simulink model "QuadrotorSimulink_w_memory_cex"  (R2020a)
settings: Solver=FixedStepAuto  StartTime=0.0  StopTime=options.T_train  FixedStep=options.dt  RelTol=1e-6
undefined symbols (not defined in the file or in its folder): options, Quad
libraries: neural x179, simulink x2
(part 7 of 10)

== system QuadrotorSimulink_w_memory_cex/NN_cex_1/Layer 2/Delays 1 ==
  "p{2}" : Inport  PortDimensions=50
      mask Display: e = 0.06;c1 = [120 230 180]/255;c2 = ([120 230 180]+0)/(256+128);c3 = ([120 230 180]+128)/(256+128);patch([0 1 1 0],[0 0 1 1],c1);patch([0 1 1 1-e 1-e 0+e],[0 0 1 1-e 0+e 0+e],c2);patch([0 0 1 1-e 0+e 0+e],[0 1 1 1-e 1-e 0+e],c3);plot([0 1 1 0 0],[0 0 1 1 0]);
  mux : Mux  Inputs=1
      mask Display: e = 0.06;c1 = [120 150 230]/255;c2 = ([120 150 230]+0)/383;c3 = ([120 150 230]+128)/383;patch([0 1 1 0],[0 0 1 1],c1);patch([0 1 1 1-e 1-e 0+e],[0 0 1 1-e 0+e 0+e],c2);patch([0 0 1 1-e 0+e 0+e],[0 1 1 1-e 1-e 0+e],c3);plot([0 1 1 0 0],[0 0 1 1 0]);disp('Mux')
  "pd{2,1}" : Outport
      mask Display: e = 0.06;c1 = [120 230 180]/255;c2 = ([120 230 180]+0)/(256+128);c3 = ([120 230 180]+128)/(256+128);patch([0 1 1 0],[0 0 1 1],c1);patch([0 1 1 1-e 1-e 0+e],[0 0 1 1-e 0+e 0+e],c2);patch([0 0 1 1-e 0+e 0+e],[0 1 1 1-e 1-e 0+e],c3);plot([0 1 1 0 0],[0 0 1 1 0]);
  wires:
  "p{2}"/1 -> mux/1
  mux/1 -> "pd{2,1}"/1

== system QuadrotorSimulink_w_memory_cex/NN_cex_1/Layer 2/LW{2,1} ==
  "ad{2,1}" : Inport  PortDimensions=50
      mask Display: e = 0.06;c1 = [120 230 180]/255;c2 = ([120 230 180]+0)/(256+128);c3 = ([120 230 180]+128)/(256+128);patch([0 1 1 0],[0 0 1 1],c1);patch([0 1 1 1-e 1-e 0+e],[0 0 1 1-e 0+e 0+e],c2);patch([0 0 1 1-e 0+e 0+e],[0 1 1 1-e 1-e 0+e],c3);plot([0 1 1 0 0],[0 0 1 1 0]);
  "IW{2,1}(1,:)'" : Constant  Value=[0.0275538326993548347842999390877594123594462871551513671875;-0.00745565907937648618408754686015527113340795040130615234375;0.66611503175745812033170523136504925787448883056640625;0.05475901990521143958279282060175319202244281768798828125;0.344437347512224933954172456651576794683933258056640625;1.1839628141689633178401663826662115752696990966796875;0.3116370266453174497911504658986814320087432861328125;0.07730669959515919231751723827983369119465351104736328125;-0.363985665723801699034112289155018515884876251220703125;0.260799759684065268761088418614235706627368927001953125;0.5559553932390013386566351982764899730682373046875;0.5868367481176670619191781952395103871822357177734375;0.443563139631132641316213494064868427813053131103515625;-0.57228815188380888212549280069652013480663299560546875;-0.4472350845444739153577984325238503515720367431640625;0.52041429315349230222409460111521184444427490234375;-1.49514504832872052730863288161344826221466064453125;3.839025236523978090730224721482954919338226318359375;-0.83636038152684888391519280048669315874576568603515625;2.770261180892548136256436919211409986019134521484375;-2.174306258179516504469575011171400547027587890625;-0.63768806122568622019031181480386294424533843994140625;-0.10146963780517899433863959757218253798782825469970703125;0.12244143511869053086993375245583592914044857025146484375;-2.7050091972379295413020372507162392139434814453125;0.033883234388811377113537304239798686467111110687255859375;-1.937067165957502279383106724708341062068939208984375;-0.02434512567339365551877250481993542052805423736572265625;-1.3585729552029144340252742040320299565792083740234375;0.0223565759681883281795311546602533780969679355621337890625;-0.030950898275129201664412903483025729656219482421875;0.340697149373347663026123655072296969592571258544921875;-0.05852572617005451227623069598848815076053142547607421875;-0.231972598769883908698119512337143532931804656982421875;-0.95302626348313912441057027535862289369106292724609375;0.08234375105086695623146653133517247624695301055908203125;-0.366614535263205587600765511524514295160770416259765625;-0.321032350030504842752776539782644249498844146728515625;0.1386987404389075084765181600232608616352081298828125;-1.410332716268217101429627291508950293064117431640625;0.3876911750625680053161659088800661265850067138671875;-0.20222266246863485061879828208475373685359954833984375;-0.6371437523569614125307225549477152526378631591796875;3.0662912359927947392179703456349670886993408203125;-0.001165993548972417588605043903271507588215172290802001953125;0.2008899619525147672849385571680613793432712554931640625;-0.06816492792016214108397065274402848444879055023193359375;-0.424260573156220399670957021953654475510120391845703125;-0.69161791521699444995618932807701639831066131591796875;0.028596534180291795224082562754119862802326679229736328125]
      mask Display: e = 0.06;c1 = [120 150 230]/255;c2 = ([120 150 230]+0)/383;c3 = ([120 150 230]+128)/383;patch([0 1 1 0],[0 0 1 1],c1);patch([0 1 1 1-e 1-e 0+e],[0 0 1 1-e 0+e 0+e],c2);patch([0 0 1 1-e 0+e 0+e],[0 1 1 1-e 1-e 0+e],c3);plot([0 1 1 0 0],[0 0 1 1 0]);disp('weights');
  "IW{2,1}(2,:)'" : Constant  Value=[-0.280572973800752134554414851663750596344470977783203125;-0.06376826585401164371180726675447658635675907135009765625;-0.93476819146209855215801098893280141055583953857421875;0.72705169346194697954643970660981722176074981689453125;-0.172177864521904255834527930346666835248470306396484375;-0.140787185209432286203679041136638261377811431884765625;0.426538355970393634475357202973100356757640838623046875;-0.289439707405152291119776464256574399769306182861328125;-0.0824665563311895166709319937581312842667102813720703125;-0.8383003997238323012908267628517933189868927001953125;-0.01928863124126110883960194541941746138036251068115234375;-0.225346299303538888381126525928266346454620361328125;0.7088162243692701647290732580586336553096771240234375;1.0224955026034676652813004693598486483097076416015625;-0.35879716511517389943008993213879875838756561279296875;0.022128490980010594169069548797779134474694728851318359375;0.5357120852447663228446117500425316393375396728515625;-0.62766932055573765314449019570020027458667755126953125;1.61542308170520332311070887953974306583404541015625;0.775974994887877134175369064905680716037750244140625;1.049763304219808457418139369110576808452606201171875;1.6714230172228912163490122111397795379161834716796875;-0.78107883860749571791615153415477834641933441162109375;0.41180896979510694944082160873222164809703826904296875;0.078029770082390204066769001656211912631988525390625;0.157969748428506029380713471255148760974407196044921875;0.06930887115900750961028364827143377624452114105224609375;-0.25182521165821059039302554083405993878841400146484375;-0.0673017608440212578013728261794312857091426849365234375;0.388768076847751664626429146665032021701335906982421875;-1.9234002406917289906829182655201293528079986572265625;0.51762869081730322751155881633167155086994171142578125;-0.07740912225261709078694138952414505183696746826171875;-0.06686671100983776483417386771179735660552978515625;0.7419276245436730032878358542802743613719940185546875;-0.13904342636608524319541402292088605463504791259765625;1.6098178034438015426843548993929289281368255615234375;-0.517302732605810167143545186263509094715118408203125;0.67228285116788677466814760919078253209590911865234375;1.420489242967595711064632268971763551235198974609375;-0.434467130876859453092464491419377736747264862060546875;0.192631001166826132386944436802878044545650482177734375;-0.127809383809272814058743961140862666070461273193359375;1.26464664389063674576618723222054541110992431640625;0.1969724906545538833935182765344507060945034027099609375;0.62756673407505469963751920658978633582592010498046875;-0.26367215443778080352643655714928172528743743896484375;-0.576491403893907516930994461290538311004638671875;-0.1502827549216607661008993090945295989513397216796875;-0.01769473689937062221844144005444832146167755126953125]
      mask Display: e = 0.06;c1 = [120 150 230]/255;c2 = ([120 150 230]+0)/383;c3 = ([120 150 230]+128)/383;patch([0 1 1 0],[0 0 1 1],c1);patch([0 1 1 1-e 1-e 0+e],[0 0 1 1-e 0+e 0+e],c2);patch([0 0 1 1-e 0+e 0+e],[0 1 1 1-e 1-e 0+e],c3);plot([0 1 1 0 0],[0 0 1 1 0]);disp('weights');
  Mux : Mux  Inputs=2
      mask Display: e = 0.06;c1 = [120 150 230]/255;c2 = ([120 150 230]+0)/383;c3 = ([120 150 230]+128)/383;patch([0 1 1 0],[0 0 1 1],c1);patch([0 1 1 1-e 1-e 0+e],[0 0 1 1-e 0+e 0+e],c2);patch([0 0 1 1-e 0+e 0+e],[0 1 1 1-e 1-e 0+e],c3);plot([0 1 1 0 0],[0 0 1 1 0]);disp('Mux');
  dotprod1 : neural/Weight Functions/dotprod
  dotprod2 : neural/Weight Functions/dotprod
  "lz{2,1}" : Outport
      mask Display: e = 0.06;c1 = [120 230 180]/255;c2 = ([120 230 180]+0)/(256+128);c3 = ([120 230 180]+128)/(256+128);patch([0 1 1 0],[0 0 1 1],c1);patch([0 1 1 1-e 1-e 0+e],[0 0 1 1-e 0+e 0+e],c2);patch([0 0 1 1-e 0+e 0+e],[0 1 1 1-e 1-e 0+e],c3);plot([0 1 1 0 0],[0 0 1 1 0]);
  wires:
  "IW{2,1}(1,:)'"/1 -> dotprod1/1
  "ad{2,1}"/1 -> dotprod1/2, dotprod2/2
  dotprod1/1 -> Mux/1
  "IW{2,1}(2,:)'"/1 -> dotprod2/1
  dotprod2/1 -> Mux/2
  Mux/1 -> "lz{2,1}"/1

== system QuadrotorSimulink_w_memory_cex/NN_online/Layer 1/Delays 1 ==
  "p{1}" : Inport  PortDimensions=20
      mask Display: e = 0.06;c1 = [120 230 180]/255;c2 = ([120 230 180]+0)/(256+128);c3 = ([120 230 180]+128)/(256+128);patch([0 1 1 0],[0 0 1 1],c1);patch([0 1 1 1-e 1-e 0+e],[0 0 1 1-e 0+e 0+e],c2);patch([0 0 1 1-e 0+e 0+e],[0 1 1 1-e 1-e 0+e],c3);plot([0 1 1 0 0],[0 0 1 1 0]);
  mux : Mux  Inputs=1
      mask Display: e = 0.06;c1 = [120 150 230]/255;c2 = ([120 150 230]+0)/383;c3 = ([120 150 230]+128)/383;patch([0 1 1 0],[0 0 1 1],c1);patch([0 1 1 1-e 1-e 0+e],[0 0 1 1-e 0+e 0+e],c2);patch([0 0 1 1-e 0+e 0+e],[0 1 1 1-e 1-e 0+e],c3);plot([0 1 1 0 0],[0 0 1 1 0]);disp('Mux')
  "pd{1,1}" : Outport
      mask Display: e = 0.06;c1 = [120 230 180]/255;c2 = ([120 230 180]+0)/(256+128);c3 = ([120 230 180]+128)/(256+128);patch([0 1 1 0],[0 0 1 1],c1);patch([0 1 1 1-e 1-e 0+e],[0 0 1 1-e 0+e 0+e],c2);patch([0 0 1 1-e 0+e 0+e],[0 1 1 1-e 1-e 0+e],c3);plot([0 1 1 0 0],[0 0 1 1 0]);
  wires:
  "p{1}"/1 -> mux/1
  mux/1 -> "pd{1,1}"/1
